simulink library "Radiation_Divison"  (R2018b)
settings: Solver=ode45  StartTime=0.0  StopTime=10.0  RelTol=1e-3  EnableMultiTasking=on
undefined symbols (not defined in the file): Germany, Potsdam
settings Model: Creator=drhf  LastModifiedBy=drhf
settings DataIOCC: LimitDataPoints=on  SaveFormat=Array  SignalLoggingSaveFormat=ModelDataLogs
settings OptimizationCC: ExpressionDepthLimit=2147483647  LifeSpan=inf
settings DebuggingCC: UnderspecifiedInitializationDetection=Classic  MergeDetectMultiDrivingBlocksExec=none  SolverPrmCheckMsg=warning  FcnCallInpInsideContextMsg=warning  StateNameClashWarn=warning  SFUnexpectedBacktrackingDiag=warning  SFNoUnconditionalDefaultTransitionDiag=warning  SFExecutionAtInitializationDiag=none
settings HardwareCC: ProdBitPerPointer=32  ProdBitPerSizeT=32  ProdBitPerPtrDiffT=32  ProdLargestAtomicFloat=None  ProdIntDivRoundTo=Undefined  ProdEndianess=Unspecified  ProdWordSize=32  ProdHWDeviceType=32-bit Generic
settings ModelReferenceCC: PropagateSignalLabelsOutOfModel=off
settings SFSimCC: SimUseLocalCustomCode=off
settings RTWCC: RTWUseLocalCustomCode=off
settings CodeAppCC: StateflowObjectComments=on
settings GRTTargetCC: TargetLangStandard=C89/C90 (ANSI)  GeneratePreprocessorConditionals=Disable all  CombineOutputUpdateFcns=off  GRTInterface=on
settings ConfigComp: CovMetricSettings=dw  CovHtmlReporting=on  CovSaveCumulativeToWorkspaceVar=on  CovSaveSingleToWorkspaceVar=on  CovExternalEMLEnable=off

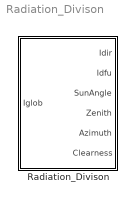
== system Radiation_Divison ==
  Radiation_Divison : Subsystem  mask(Radiation Division){latitude=52.393800 % Potsdam / Germany, longitude=-13.065100 % Potsdam, longitude0=-15  % CET}
      mask prompts: latitude "Latitude [-90;90], north positive"; longitude "Longitude  [-180;180], west positive"; longitude0 "reference longitude (timezone)"
      mask help:
      | Calculates the direct and diffusive radiation on the horizontal surface as parts of the global radiation.
      |
      | INPUT VECTOR:
      |   time      : real time or simulation time  [s]
      |   Iglob     : global radiation on horizontal surface (W/m²)
      |
      | OUTPUT VECTORS:
      |   Idir           : direct radiation (W/m²)
      |   Idfu          : diffusive radiation (W/m²)
      |   SunAngle
      |   Zenith
      |   Azimuth
      mask Help: web(fullfile(path_carnot('help'),'Radiation_Divison.html'),'-helpbrowser')

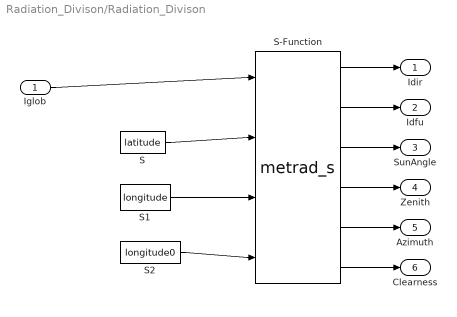
== system Radiation_Divison/Radiation_Divison ==
  Iglob : Inport
  S : Constant  Value=latitude
  S-Function : S-Function  FunctionName=metrad_s  SFunctionDeploymentMode=off  EnableBusSupport=off
  S1 : Constant  Value=longitude
  S2 : Constant  Value=longitude0
  Idir : Outport
  Idfu : Outport  Port=2
  SunAngle : Outport  Port=3
  Zenith : Outport  Port=4
  Azimuth : Outport  Port=5
  Clearness : Outport  Port=6
  wires:
  S-Function/6 -> Clearness/1
  S-Function/5 -> Azimuth/1
  S-Function/4 -> Zenith/1
  S-Function/3 -> SunAngle/1
  S-Function/2 -> Idfu/1
  S-Function/1 -> Idir/1
  Iglob/1 -> S-Function/1
  S/1 -> S-Function/2
  S1/1 -> S-Function/3
  S2/1 -> S-Function/4
